simulink model "P3_SIM"  (R2024b)
settings: Solver=ode4  StartTime=0.0  StopTime=T_SIM  FixedStep=T_s  RelTol=1e-3
values from neighbouring files (symbols this model uses):
  D = diag([0.001, 0.001, 0.0175/6, 0.0175/6, 0.0175/6, 0.0175/6*T_s, 0.0175/6*T_s].^2)    [P3_script_FIXED.m]    (also in part3_results.mat = [1e-06 0 0 0 0 0 0 0 1e-06 0 0 0 ... (49 elements, 7x7)])
  d = 0.18428    [P3_script_FIXED.m]    (also in part3_results.mat)
  d_id = 0.18428    [P3_script_FIXED.m]    (also in part3_results.mat)
  H_enc = [0, 0, 0, 1, 0, 0, 0 ... (first row only)    [P3_script_FIXED.m]    (also in part3_results.mat = [0 0 0 0 0 0 1 0 0 1 0 0 ... (14 elements, 2x7)])
  H_gyro = [0, 0, 0, 0, 0, -r_id/d_id, r_id/d_id]    [P3_script_FIXED.m]    (also in part3_results.mat = [0 0 0 0 0 -0.179943564142 0.179943564142])
  H_motion_cap = [1, 0, 0, 0, 0, 0, 0 ... (first row only)    [P3_script_FIXED.m]    (also in part3_results.mat = [1 0 0 0 1 0 0 0 1 0 0 0 ... (21 elements, 3x7)])
  omega_max = 10    [P3_script_FIXED.m]    (also in part3_results.mat)
  P_INIT_EKF = diag([0.001, 0.001, 0.0175/6, 0.0175/6, 0.0175/6, 0.0175/6*T_s, 0.0175/6*T_s].^2)    [P3_script_FIXED.m]    (also in part3_results.mat = [1e-06 0 0 0 0 0 0 0 1e-06 0 0 0 ... (49 elements, 7x7)])
  p_loss = sim_output.p_loss.signals.values(1)    [P3_save_data.m]    (also in P3_script_FIXED.m = p_loss_values(i); part3_results.mat = 0)
  PHI_INIT = [0;0]    [P3_script_FIXED.m]    (also in part3_results.mat = [0 0])
  Q_INIT = q(:,1)    [P3_script_FIXED.m]    (also in part3_results.mat = [-0.5 -0.5 1.57079632679])
  Q_INIT_LOC = Q_INIT    [P3_script_FIXED.m]    (also in part3_results.mat = [-0.5 -0.5 1.57079632679])
  r = 0.03316    [P3_script_FIXED.m]    (also in part3_results.mat)
  R_3 = diag(([var_motion_capture, var_motion_capture, var_motion_capture,               ENCODER_QUANTIZATION/6, ENCODER_QUANTIZATION/6, var_IMU]).^2)    [P3_script_FIXED.m]    (also in part3_results.mat = [1e-06 0 0 0 0 0 0 1e-06 0 0 0 0 ... (36 elements, 6x6)])
  r_id = 0.03316    [P3_script_FIXED.m]    (also in part3_results.mat)
  T_s = (sim_output.tout(end)-sim_output.tout(1))/(length(sim_output.tout)-1)    [P3_save_data.m]    (also in P3_script_FIXED.m = 0.04; part3_results.mat = 0.04)
  Z_INIT_EKF = [Q_INIT; 0; 0; 0; 0]    [P3_script_FIXED.m]    (also in part3_results.mat = [-0.5 -0.5 1.57079632679 0 0 0 0])
undefined symbols (not defined in the file or in its folder): Ts, X, Y
libraries: robotlib x11, sharedtransform x1
settings Model: Creator=tomailoren  LastModifiedBy=tomailoren
settings OptimizationCC: DefaultParameterBehavior=Inlined  EnhancedBackFolding=on  PassReuseOutputArgsAs=Individual arguments  ZeroExternalMemoryAtStartup=off  ZeroInternalMemoryAtStartup=off  MaxStackSize=64  OptimizeBlockOrder=speed  DifferentSizesBufferReuse=on  OptimizationCustomize=off  EfficientTunableParamExpr=on
settings DebuggingCC: ParameterTunabilityLossMsg=error
settings HardwareCC: ProdBitPerPointer=32  ProdBitPerSizeT=32  ProdBitPerPtrDiffT=32  ProdLargestAtomicFloat=None  ProdIntDivRoundTo=Undefined  ProdEndianess=Unspecified  ProdWordSize=32  ProdHWDeviceType=Generic->Unspecified (assume 32-bit Generic)
settings SFSimCC: MATLABDynamicMemAlloc=off
settings RTWCC: Description=Embedded Coder  SystemTargetFile=ert.tlc  HardwareBoard=Robot Operating System (ROS)  TLCOptions="-aInlineSetEventsForThisBaseRateFcn=TLC_FALSE -aSuppressMultiTaskScheduler=TLC_FALSE  -aRateBasedStepFcn=0"  TemplateMakefile=ert_default_tmf  Toolchain=Catkin  TargetLang=C++
settings CodeAppCC: ForceParamTrailComments=on  IgnoreCustomStorageClasses=off  OperatorAnnotations=on  SimulinkDataObjDesc=on  SFDataObjDesc=on  InsertBlockDesc=on

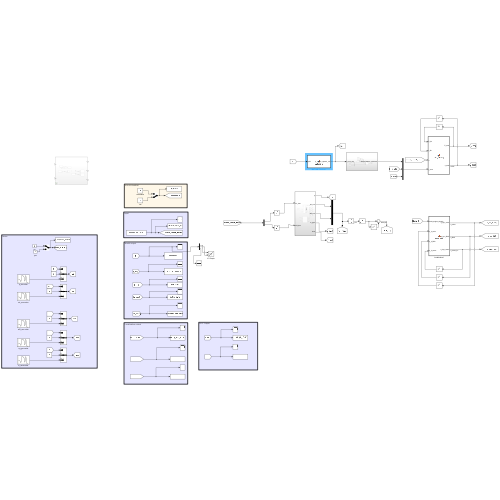
[thumbnail: Simulink's stored preview of the top-level diagram]
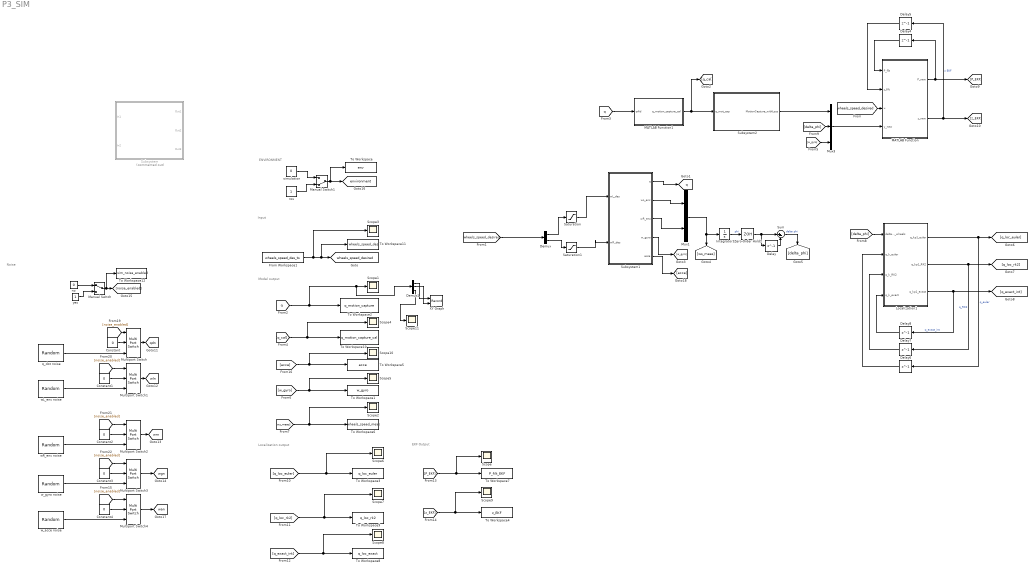
== system P3_SIM ==
  note: ENVIRONMENT
  note: Noise
  note: EKF Output
  note: Localization output
  note: Model output
  note: Input
  Constant{,1..4} (5 alike) : Constant  Value=0
  Delay : Delay  DelayLength=1  InitialCondition=[0;0]  SampleTime=T_s
  Delay4 : Delay  DelayLength=1  InitialCondition=P_INIT_EKF  SampleTime=T_s
  Delay5 : Delay  DelayLength=1  InitialCondition=Z_INIT_EKF  SampleTime=T_s
  Delay6 : Delay  DelayLength=1  InitialCondition=Q_INIT_LOC
  Delay7 : Delay  DelayLength=1  InitialCondition=Q_INIT_LOC
  Delay8 : Delay  DelayLength=1  InitialCondition=Q_INIT_LOC
  Demux : Demux  Outputs=2
  Demux1 : Demux  Outputs=3
  From Workspace1 : FromWorkspace  VariableName=wheels_speed_des_ts
  Integrator5 : Integrator  InitialCondition=PHI_INIT
  Localization1 : MATLAB Function  TreatAsAtomicUnit=on
  MATLAB Function : MATLAB Function  TreatAsAtomicUnit=on
  MATLAB Function1 : MATLAB Function  TreatAsAtomicUnit=on
  Manual Switch : ManualSwitch
  Manual Switch1 : ManualSwitch  CurrentSetting=0
  Multiport Switch{,1..4} (5 alike) : MultiPortSwitch  DataPortOrder=Zero-based contiguous  Inputs=2  zeroidx=on  SaturateOnIntegerOverflow=off  InputSameDT=off
  Mux1 : Mux  Inputs=2
  Mux3 : Mux  Inputs=3
  Saturation : Saturate  UpperLimit=omega_max  LowerLimit=-omega_max
  Saturation1 : Saturate  UpperLimit=omega_max  LowerLimit=-omega_max
  Scope{,1..11} (12 alike) : Scope
  Subsystem : Subsystem  Commented=on
  Subsystem1 : Subsystem
  Subsystem2 : Subsystem
  Sum : Sum  Inputs=|+-
  To Workspace : ToWorkspace  VariableName=env  SaveFormat=Structure  SampleTime=-1
      settings: Save2DSignal=2-D array (concatenate along first dimension)
  To Workspace1 : ToWorkspace  VariableName=w_gyro  SaveFormat=Structure With Time  SampleTime=-1
  To Workspace10 : ToWorkspace  VariableName=q_motion_capture_cal  SaveFormat=Structure With Time  SampleTime=-1
  To Workspace11 : ToWorkspace  VariableName=wheels_speed_des  SaveFormat=Structure With Time  SampleTime=-1
  To Workspace12 : ToWorkspace  VariableName=sim_noise_enabled  SaveFormat=Structure  SampleTime=-1
      settings: Save2DSignal=2-D array (concatenate along first dimension)
  To Workspace2 : ToWorkspace  VariableName=q_motion_capture  SaveFormat=Structure With Time  SampleTime=-1
  To Workspace3 : ToWorkspace  VariableName=q_loc_euler  SaveFormat=Structure With Time  SampleTime=-1
  To Workspace4 : ToWorkspace  VariableName=z_EKF  SaveFormat=Structure With Time  SampleTime=-1
  To Workspace5 : ToWorkspace  VariableName=acce  SaveFormat=Structure With Time  SampleTime=-1
  To Workspace6 : ToWorkspace  VariableName=wheels_speed_meas  SaveFormat=Structure With Time  SampleTime=-1
  To Workspace7 : ToWorkspace  VariableName=P_filt_EKF  SaveFormat=Structure With Time  SampleTime=-1
  To Workspace8 : ToWorkspace  VariableName=q_loc_exact  SaveFormat=Structure With Time  SampleTime=-1
  To Workspace9 : ToWorkspace  VariableName=q_loc_rk2  SaveFormat=Structure With Time  SampleTime=-1
  XY Graph : Record  FileSettingsInternal="{\"entries\":[{\"content\":{\"excelSettings\":{\"content\":{},\"type\":\"Streamout.ExcelSettings\"}},\"type\":\"Streamout.FileSettingStorage\",\"uuid\":\"\"}],\"packageUris\":[\"http:\\/\\/schema.mathworks.com\\/mf0\\/streamout_blocks\\/R2020a\"],\"version\":\"1.0\"}"  Layout=[1 1]  SignalsInternal="{\"entries\":[{\"content\":{\"signals\":[{\"content\":{\"blockPath\":[],\"dimensions\":[1,1],\"domain\":\"\",\"lineColor\":\"#a2142f\",\"plots\":[ 1 ],\"port\":1,\"sid\":[\"\"],\"signalID\":1,\"signalName\":\"Demux1:1\"},\"type\":\"RecordBlkView.Signal\",\"uuid\":\"\"},{\"content\":{\"blockPath\":[],\"dimensions\":[1,1],\"domain\":\"\",\"lineColor\":\"#139fff\",\"plots\":[ 1 ],\"port\":2,\"sid\":[\"\"],\"signalID\":2,\"signalName\":\"Demux1:2\"},\"type\":\"RecordBlkView.Signal\",\"uuid\":\"\"}]},\"type\":\"RecordBlkView.InputSignals\",\"uuid\":\"\"}],\"packageUris\":[\"http:\\/\\/schema.mathworks.com\\/mf0\\/streamout_blocks\\/R2020a\"],\"version\":\"1.0\"}"  VisualizationBindings="{\"xyplotplugin\":{\"info\":[{\"series\":[{\"bindingParametersList\":[{\"parameter\":\"X-Axis\",\"signalID\":1,\"signalName\":\"Demux1:1\"},{\"parameter\":\"Y-Axis\",\"signalID\":2,\"signalName\":\"Demux1:2\"}],\"seriesID\":0}],\"subplotID\":1}]}}"  CompatibilityTag=XY
  Zero-Order Hold1 : ZeroOrderHold  SampleTime=T_s
  no : Constant  Value=0
  q_dot noise : RandomNumber  SampleTime=T_s
  ros : Constant
  simulation : Constant  Value=0
  wL_enc noise : RandomNumber  Variance=0.25  Seed=1  SampleTime=T_s
  wR_enc noise : RandomNumber  Variance=0.25  Seed=2  SampleTime=T_s
  w_acce noise : RandomNumber  Variance=0.01  Seed=3  SampleTime=T_s
  w_gyro noise : RandomNumber  Variance=0.01  Seed=3  SampleTime=T_s
  yes : Constant
  tag scope: environment=global, q=global, qdn=global, wan=global, wgn=global, wheels_speed_desired=global, wln=global, wrn=global
  wires:
  Mux1/1 -> Integrator5/1, [ws_meas]
  Zero-Order Hold1/1 -> Delay/1, Sum/1
  Delay/1 -> Sum/2
  Integrator5/1 -> Zero-Order Hold1/1  "phi"
  Demux/1 -> Saturation/1
  Demux/2 -> Saturation1/1
  [wheels_speed_desired] -> Demux/1
  Delay5/1 -> MATLAB Function/2(z_filt)
  MATLAB Function/2(z_new) -> [z_EKF], Delay5/1  "z EKF"
  Delay4/1 -> MATLAB Function/1(P_filt)
  MATLAB Function/1(P_new) -> [P_EKF], Delay4/1
  Localization1/3(q_kp1_exact) -> [q_exact_int], Delay8/1  "q_exact_int"
  Localization1/1(q_kp1_euler) -> [q_loc_euler], Delay6/1  "q_euler"
  Delay6/1 -> Localization1/2(q_k_euler)
  Localization1/2(q_kp1_RK2) -> [q_loc_rk2], Delay7/1  "q_RK2"
  Delay8/1 -> Localization1/4(q_k_exact)
  Delay7/1 -> Localization1/3(q_k_RK2)
  Subsystem2/1(MotionCapture_withLoss) -> Mux3/1
  Mux3/1 -> MATLAB Function/4(y_new)
  MATLAB Function1/1(q_motion_capture_cal) -> [q_cal], Subsystem2/1(q_mot_cap)
  [wheels_speed_desired] -> MATLAB Function/3(u)
  From Workspace1/1 -> Scope3/1, To Workspace11/1, [wheels_speed_desired]
  [q] -> MATLAB Function1/1(q4id)
  [q_cal] -> To Workspace10/1, Scope4/1
  [w_gyro] -> Mux3/3
  [w_gyro] -> Scope5/1, To Workspace1/1
  [ws_meas] -> Scope2/1, To Workspace6/1
  Sum/1 -> [delta_phi]  "delta phi"
  [delta_phi] -> Localization1/1(delta_angles_wheels)
  [delta_phi] -> Mux3/2
  [q_loc_euler] -> Scope6/1, To Workspace3/1
  [q_loc_rk2] -> Scope7/1, To Workspace9/1
  [q_exact_int] -> Scope8/1, To Workspace8/1
  [P_EKF] -> Scope/1, To Workspace7/1
  [z_EKF] -> Scope9/1, To Workspace4/1
  Subsystem1/4(w_gyro) -> [w_gyro]
  Subsystem1/2(wL_enc) -> Mux1/1
  Subsystem1/3(wR_enc) -> Mux1/2
  yes/1 -> Manual Switch/2
  no/1 -> Manual Switch/1
  Manual Switch/1 -> To Workspace12/1, [noise_enabled]
  Multiport Switch/1 -> [qdn]
  [noise_enabled] -> Multiport Switch/1
  q_dot noise/1 -> Multiport Switch/3
  Constant/1 -> Multiport Switch/2
  [noise_enabled] -> Multiport Switch1/1
  Constant1/1 -> Multiport Switch1/2
  wL_enc noise/1 -> Multiport Switch1/3
  Multiport Switch1/1 -> [wln]
  [noise_enabled] -> Multiport Switch2/1
  Constant2/1 -> Multiport Switch2/2
  wR_enc noise/1 -> Multiport Switch2/3
  Multiport Switch2/1 -> [wrn]
  [noise_enabled] -> Multiport Switch3/1
  Constant3/1 -> Multiport Switch3/2
  Multiport Switch3/1 -> [wgn]
  w_gyro noise/1 -> Multiport Switch3/3
  Saturation/1 -> Subsystem1/1(wL_des)
  Saturation1/1 -> Subsystem1/2(wR_des)
  simulation/1 -> Manual Switch1/1
  ros/1 -> Manual Switch1/2
  Subsystem1/1(q) -> [q]
  Manual Switch1/1 -> To Workspace/1, [environment]
  Constant4/1 -> Multiport Switch4/2
  Multiport Switch4/1 -> [wan]
  w_acce noise/1 -> Multiport Switch4/3
  [noise_enabled] -> Multiport Switch4/1
  Subsystem1/5(acce) -> [acce]
  [acce] -> Scope10/1, To Workspace5/1
  [q] -> Demux1/1, Scope1/1, To Workspace2/1
  Demux1/3 -> Scope11/1
  Demux1/2 -> XY Graph/2
  Demux1/1 -> XY Graph/1

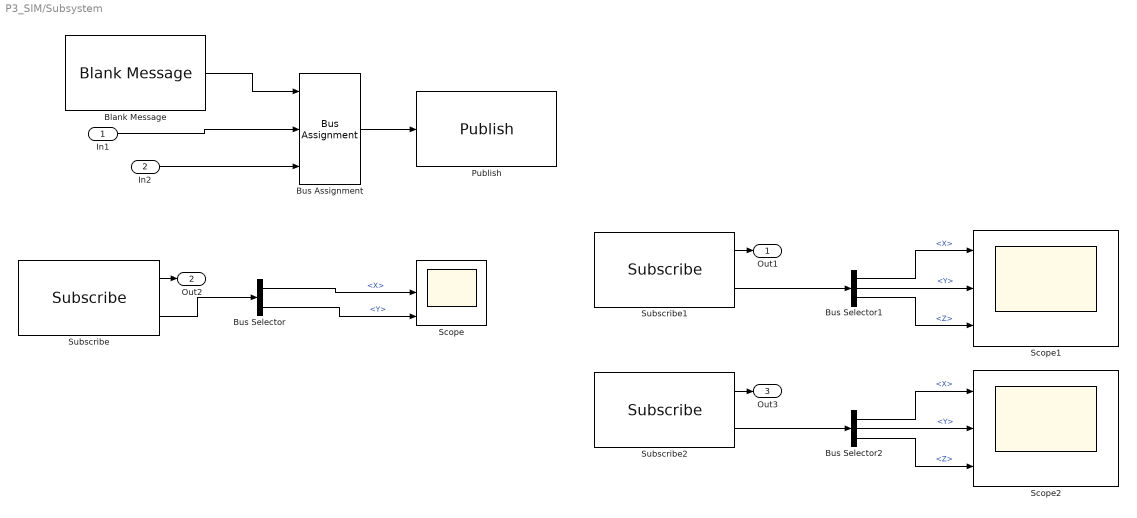
== system P3_SIM/Subsystem ==
  In1 : Inport
  In2 : Inport  Port=2
  Blank Message : robotlib/Blank Message  messageClass=Message  entityType=geometry_msgs/Vector3  messageType=geometry_msgs/Vector3  SampleTime=Ts  legacyBusStruct=off
  Bus Assignment : BusAssignment  AssignedSignals=X,Y
  Bus Selector : BusSelector  OutputSignals=X,Y
  Bus Selector1 : BusSelector  OutputSignals=X,Y,Z
  Bus Selector2 : BusSelector  OutputSignals=X,Y,Z
  Publish : robotlib/Publish  topicSource=Select from ROS network  topic=/turtlebot_01/cmd_wheels  messageType=geometry_msgs/Vector3  legacyBusStruct=off  messageQueueLength=1
  Scope : Scope  NumInputPorts=3
  Scope1 : Scope  NumInputPorts=3
  Scope2 : Scope  NumInputPorts=3
  Subscribe : robotlib/Subscribe  topicSource=Select from ROS network  topic=/turtlebot_01/wheelSpeeds  messageType=geometry_msgs/Vector3  SampleTime=Ts  legacyBusStruct=off  messageQueueLength=1
  Subscribe1 : robotlib/Subscribe  topicSource=Select from ROS network  topic=/turtlebot_01/gyroscope  messageType=geometry_msgs/Vector3  SampleTime=Ts  legacyBusStruct=off  messageQueueLength=1
  Subscribe2 : robotlib/Subscribe  topicSource=Select from ROS network  topic=/turtlebot_01/accelerometer  messageType=geometry_msgs/Vector3  SampleTime=Ts  legacyBusStruct=off  messageQueueLength=1
  Out1 : Outport
  Out2 : Outport  Port=2
  Out3 : Outport  Port=3
  wires:
  Bus Selector1/2 -> Scope1/2  "<Y>"
  Subscribe/2 -> Bus Selector/1
  Bus Selector2/1 -> Scope2/1  "<X>"
  Bus Selector1/3 -> Scope1/3  "<Z>"
  Bus Selector2/2 -> Scope2/2  "<Y>"
  Subscribe1/1 -> Out1/1
  Bus Assignment/1 -> Publish/1
  Bus Selector1/1 -> Scope1/1  "<X>"
  Bus Selector/1 -> Scope/2  "<X>"
  In2/1 -> Bus Assignment/3
  Subscribe1/2 -> Bus Selector1/1
  Subscribe2/2 -> Bus Selector2/1
  Blank Message/1 -> Bus Assignment/1
  Bus Selector/2 -> Scope/3  "<Y>"
  Bus Selector2/3 -> Scope2/3  "<Z>"
  In1/1 -> Bus Assignment/2
  Subscribe2/1 -> Out3/1
  Subscribe/1 -> Out2/1

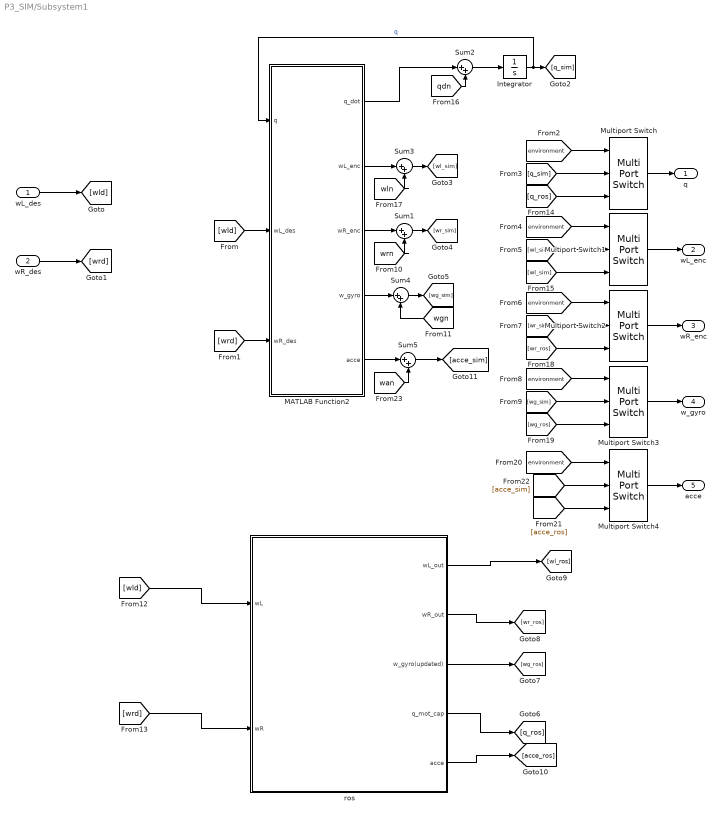
== system P3_SIM/Subsystem1 ==
  wL_des : Inport
  wR_des : Inport  Port=2
  Integrator : Integrator  InitialCondition=Q_INIT
  MATLAB Function2 : MATLAB Function  TreatAsAtomicUnit=on
  Multiport Switch{,1..4} (5 alike) : MultiPortSwitch  DataPortOrder=Zero-based contiguous  Inputs=2  zeroidx=on  SaturateOnIntegerOverflow=off  InputSameDT=off
  Sum{1..5} (5 alike) : Sum  Inputs=|++
  ros : Subsystem
  q : Outport
  wL_enc : Outport  Port=2
  wR_enc : Outport  Port=3
  w_gyro : Outport  Port=4
  acce : Outport  Port=5
  wires:
  Sum2/1 -> Integrator/1
  Integrator/1 -> [q_sim], MATLAB Function2/1(q)  "q"
  [qdn] -> Sum2/2
  MATLAB Function2/1(q_dot) -> Sum2/1
  wL_des/1 -> [wld]
  wR_des/1 -> [wrd]
  [wld] -> MATLAB Function2/2(wL_des)
  [wrd] -> MATLAB Function2/3(wR_des)
  [environment] -> Multiport Switch/1
  [q_sim] -> Multiport Switch/2
  Multiport Switch/1 -> q/1
  [environment] -> Multiport Switch1/1
  [wl_sim] -> Multiport Switch1/2
  Multiport Switch1/1 -> wL_enc/1
  [environment] -> Multiport Switch2/1
  [wr_sim] -> Multiport Switch2/2
  Multiport Switch2/1 -> wR_enc/1
  [environment] -> Multiport Switch3/1
  [wg_sim] -> Multiport Switch3/2
  Multiport Switch3/1 -> w_gyro/1
  [wln] -> Sum3/2
  Sum3/1 -> [wl_sim]
  MATLAB Function2/2(wL_enc) -> Sum3/1
  [wrn] -> Sum1/2
  MATLAB Function2/3(wR_enc) -> Sum1/1
  Sum1/1 -> [wr_sim]
  [wgn] -> Sum4/2
  MATLAB Function2/4(w_gyro) -> Sum4/1
  Sum4/1 -> [wg_sim]
  [q_ros] -> Multiport Switch/3
  [wl_sim] -> Multiport Switch1/3
  [wr_ros] -> Multiport Switch2/3
  [wg_ros] -> Multiport Switch3/3
  Multiport Switch4/1 -> acce/1
  [environment] -> Multiport Switch4/1
  [acce_sim] -> Multiport Switch4/2
  [acce_ros] -> Multiport Switch4/3
  MATLAB Function2/5(acce) -> Sum5/1
  Sum5/1 -> [acce_sim]
  [wan] -> Sum5/2
  ros/1(wL_out) -> [wl_ros]
  ros/2(wR_out) -> [wr_ros]
  ros/5(acce) -> [acce_ros]
  ros/4(q_mot_cap) -> [q_ros]
  ros/3(w_gyro(updated)) -> [wg_ros]
  [wld] -> ros/1(wL)
  [wrd] -> ros/2(wR)

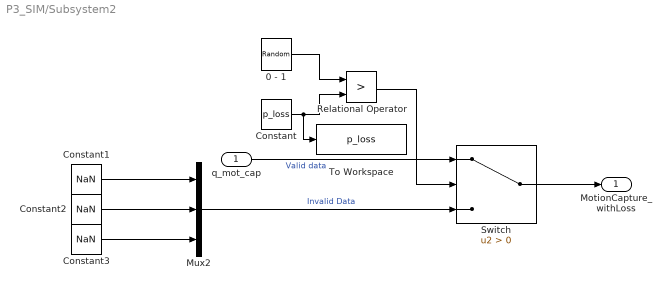
== system P3_SIM/Subsystem2 ==
  q_mot_cap : Inport
  0 - 1 : UniformRandomNumber  Minimum=0  SampleTime=T_s
  Constant : Constant  Value=p_loss
  Constant1 : Constant  Value=NaN
  Constant2 : Constant  Value=NaN
  Constant3 : Constant  Value=NaN
  Mux2 : Mux  Inputs=3
  Relational Operator : RelationalOperator  Operator=>  OutDataTypeStr=boolean  RndMeth=Simplest  InputSameDT=off
  Switch : Switch  Criteria=u2 > Threshold  SaturateOnIntegerOverflow=off  InputSameDT=off
  To Workspace : ToWorkspace  VariableName=p_loss  SaveFormat=Structure  SampleTime=-1
      settings: Save2DSignal=2-D array (concatenate along first dimension)
  MotionCapture_withLoss : Outport
  wires:
  0 - 1/1 -> Relational Operator/1
  Constant/1 -> To Workspace/1, Relational Operator/2
  Switch/1 -> MotionCapture_withLoss/1
  Relational Operator/1 -> Switch/2
  Constant2/1 -> Mux2/2
  Mux2/1 -> Switch/3  "Invalid Data"
  Constant1/1 -> Mux2/1
  q_mot_cap/1 -> Switch/1  "Valid data"
  Constant3/1 -> Mux2/3

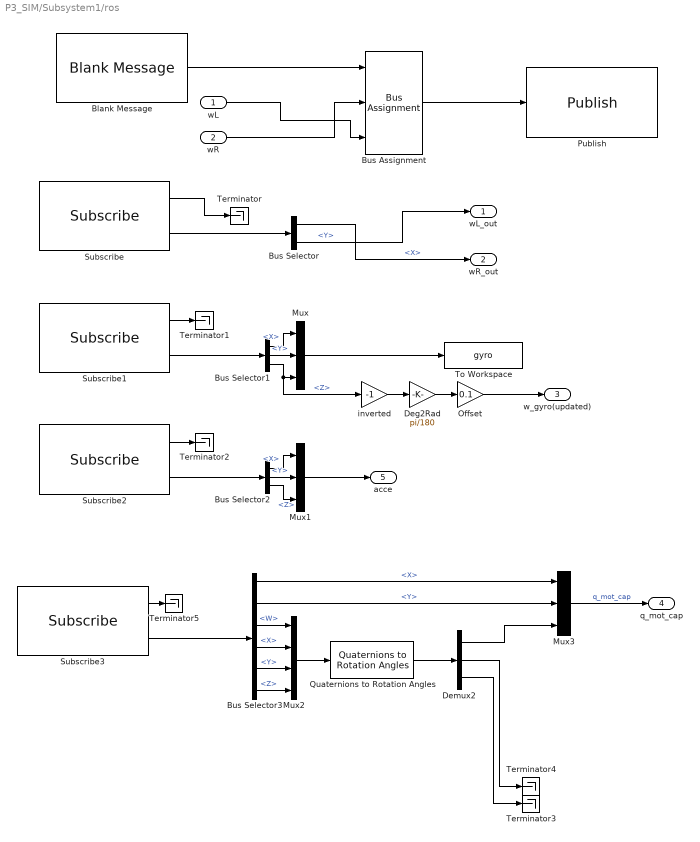
== system P3_SIM/Subsystem1/ros ==
  wL : Inport
  wR : Inport  Port=2
  Blank Message : robotlib/Blank Message  messageClass=Message  entityType=geometry_msgs/Vector3  messageType=geometry_msgs/Vector3  SampleTime=T_s  legacyBusStruct=off
  Bus Assignment : BusAssignment  AssignedSignals=X,Y
  Bus Selector : BusSelector  OutputSignals=X,Y
  Bus Selector1 : BusSelector  OutputSignals=X,Y,Z
  Bus Selector2 : BusSelector  OutputSignals=X,Y,Z
  Bus Selector3 : BusSelector  OutputSignals=Pose.Pose.Position.X,Pose.Pose.Position.Y,Pose.Pose.Orientation.W,Pose.Pose.Orientation.X,Pose.Pose.Orientation.Y,Pose.Pose.Orientation.Z
  Deg2Rad : Gain  Gain=pi/180
  Demux2 : Demux  Outputs=3
  Mux : Mux  Inputs=3
  Mux1 : Mux  Inputs=3
  Mux2 : Mux
  Mux3 : Mux  Inputs=3
  Offset : Gain  Gain=0.1
  Publish : robotlib/Publish  topicSource=Select from ROS network  topic=/turtlebot_01/cmd_wheels  messageType=geometry_msgs/Vector3  legacyBusStruct=off  messageQueueLength=1
  Quaternions to Rotation Angles : sharedtransform/Quaternions to Rotation Angles  rotationOrder=ZYX  aMode=aMode
  Subscribe : robotlib/Subscribe  topicSource=Select from ROS network  topic=/turtlebot_01/wheelSpeeds  messageType=geometry_msgs/Vector3  SampleTime=T_s  legacyBusStruct=off  messageQueueLength=1
  Subscribe1 : robotlib/Subscribe  topicSource=Select from ROS network  topic=/turtlebot_01/gyroscope  messageType=geometry_msgs/Vector3  SampleTime=T_s  legacyBusStruct=off  messageQueueLength=1
  Subscribe2 : robotlib/Subscribe  topicSource=Select from ROS network  topic=/turtlebot_01/accelerometer  messageType=geometry_msgs/Vector3  SampleTime=T_s  legacyBusStruct=off  messageQueueLength=1
  Subscribe3 : robotlib/Subscribe  topicSource=Select from ROS network  topic=/turtlebot_01/odom  messageType=nav_msgs/Odometry  SampleTime=T_s  legacyBusStruct=off  messageQueueLength=1
  Terminator{,1..5} (6 alike) : Terminator
  To Workspace : ToWorkspace  VariableName=gyro  SaveFormat=Structure With Time  SampleTime=-1
  inverted : Gain  Gain=-1
  wL_out : Outport
  wR_out : Outport  Port=2
  w_gyro(updated) : Outport  Port=3
  q_mot_cap : Outport  Port=4
  acce : Outport  Port=5
  wires:
  Subscribe2/2 -> Bus Selector2/1
  Bus Selector3/6 -> Mux2/4  "<Z>"
  Mux3/1 -> q_mot_cap/1  "q_mot_cap"
  wR/1 -> Bus Assignment/2
  Bus Selector/1 -> wR_out/1  "<X>"
  Bus Selector1/2 -> Mux/2  "<Y>"
  Bus Selector2/2 -> Mux1/2  "<Y>"
  Bus Selector2/1 -> Mux1/1  "<X>"
  Bus Assignment/1 -> Publish/1
  Subscribe2/1 -> Terminator2/1
  Demux2/2 -> Terminator4/1
  Mux2/1 -> Quaternions to Rotation Angles/1
  inverted/1 -> Deg2Rad/1
  Bus Selector3/4 -> Mux2/2  "<X>"
  Bus Selector3/1 -> Mux3/1  "<X>"
  Subscribe3/1 -> Terminator5/1
  Subscribe/2 -> Bus Selector/1
  Mux1/1 -> acce/1
  Deg2Rad/1 -> Offset/1
  Bus Selector3/5 -> Mux2/3  "<Y>"
  Quaternions to Rotation Angles/1 -> Demux2/1
  Bus Selector1/3 -> inverted/1, Mux/3  "<Z>"
  Demux2/3 -> Terminator3/1
  Demux2/1 -> Mux3/3
  Offset/1 -> w_gyro(updated)/1
  wL/1 -> Bus Assignment/3
  Bus Selector3/3 -> Mux2/1  "<W>"
  Bus Selector1/1 -> Mux/1  "<X>"
  Subscribe3/2 -> Bus Selector3/1
  Bus Selector2/3 -> Mux1/3  "<Z>"
  Mux/1 -> To Workspace/1
  Subscribe/1 -> Terminator/1
  Bus Selector/2 -> wL_out/1  "<Y>"
  Subscribe1/2 -> Bus Selector1/1
  Subscribe1/1 -> Terminator1/1
  Blank Message/1 -> Bus Assignment/1
  Bus Selector3/2 -> Mux3/2  "<Y>"

== matlab function P3_SIM/Localization1 ==
  data: delta_angles_wheels input; q_k_euler input; q_k_RK2 input; q_k_exact input; r_id parameter; d_id parameter; q_kp1_euler output; T_s parameter; q_kp1_RK2 output; q_kp1_exact output
function [q_kp1_euler, q_kp1_RK2, q_kp1_exact] = localization(delta_angles_wheels, q_k_euler, q_k_RK2, q_k_exact, r_id, d_id, T_s)

    r = r_id;
    d = d_id;

    % extraction data
    delta_phi_L = delta_angles_wheels(1);
    delta_phi_R = delta_angles_wheels(2);

    x_k_euler = q_k_euler(1); 
    y_k_euler = q_k_euler(2); 
    theta_k_euler = q_k_euler(3);
    
    x_k_RK2 = q_k_RK2(1); 
    y_k_RK2 = q_k_RK2(2); 
    theta_k_RK2 = q_k_RK2(3);

    x_k_exact = q_k_exact(1);
    y_k_exact = q_k_exact(2); 
    theta_k_exact = q_k_exact(3);


    % velocities estimate
    v_k = r / (2*T_s) * (delta_phi_R + delta_phi_L);
    w_k = r / (d*T_s) * (delta_phi_R - delta_phi_L);
    
    % Euler integration
    x_kp1_euler = x_k_euler + v_k * T_s * cos(theta_k_euler);
    y_kp1_euler = y_k_euler + v_k * T_s * sin(theta_k_euler);
    theta_kp1_euler = theta_k_euler + w_k * T_s;
    
    q_kp1_euler = [x_kp1_euler; y_kp1_euler; theta_kp1_euler];
    
    % RK2 Integration
    x_kp1_RK2 = x_k_RK2 + v_k * T_s * cos(theta_k_RK2 + (w_k * T_s)/2);
    y_kp1_RK2 = y_k_RK2 + v_k * T_s * sin(theta_k_RK2 + (w_k * T_s)/2);
    theta_kp1_RK2 = theta_k_RK2 + w_k * T_s;
    
    q_kp1_RK2 = [x_kp1_RK2; y_kp1_RK2; theta_kp1_RK2];
    
    % Exact Integration
    if abs(w_k) < 1e-4
        % use RK2 approximation to avoid division by zero when w_k is near 0
        x_kp1_exact = x_k_exact + v_k * T_s * cos(theta_k_exact + (w_k * T_s)/2);
        y_kp1_exact = y_k_exact + v_k * T_s * sin(theta_k_exact + (w_k * T_s)/2);
    else
        % Exact formulas
        x_kp1_exact = x_k_exact + (v_k / w_k) * (sin(theta_k_exact + w_k * T_s) - sin(theta_k_exact));
        y_kp1_exact = y_k_exact - (v_k / w_k) * (cos(theta_k_exact + w_k * T_s) - cos(theta_k_exact));
    end
    theta_kp1_exact = theta_k_exact + w_k * T_s;
    
    q_kp1_exact = [x_kp1_exact; y_kp1_exact; theta_kp1_exact];
    
end

== matlab function P3_SIM/MATLAB Function1 ==
  data: q4id input; q_motion_capture_cal output
function q_motion_capture_cal = calibration(q4id)

x_off_cal = -0.00434;
y_off_cal = -0.00361;
theta_off = 0.02331;


theta_cal = q4id(3) - theta_off;
x_cal = q4id(1) - (x_off_cal * cos(theta_cal) - y_off_cal * sin(theta_cal));
y_cal = q4id(2) - (x_off_cal * sin(theta_cal) + y_off_cal * cos(theta_cal));


q_motion_capture_cal = [x_cal; y_cal; theta_cal];

== matlab function P3_SIM/Subsystem1/MATLAB Function2 ==
  data: q input; q_dot output; wL_des input; wR_des input; wL_enc output; wR_enc output; w_gyro output; r parameter; d parameter; T_s parameter; acce output
function [q_dot, wL_enc, wR_enc, w_gyro, acce] = robot_simulator(q, wL_des, wR_des, r, d, T_s)
    
    wL_enc = wL_des;
    wR_enc = wR_des;
      
    v = (r/2) * (wR_des + wL_des);
    omega = (r/d) * (wR_des - wL_des);
    
    w_gyro = -omega;
    
    q_dot= zeros(3,1);
    
    q_dot(1) = v*cos(q(3));
    q_dot(2) = v*sin(q(3));
    q_dot(3) = omega;

    acce = [0;0;0];
    
end

== matlab function P3_SIM/MATLAB Function ==
  data: P_filt input; P_new output; z_filt input; z_new output; u input; y_new input; D parameter; T_s parameter; r_id parameter; d_id parameter; H_enc parameter; H_gyro parameter; H_motion_cap parameter; R_3 parameter
function [P_new, z_new] = EKF_filtering(P_filt, z_filt, u, y_new, D, T_s, r_id, d_id, H_enc, H_gyro, H_motion_cap, R_3)

    % Def state z_filt: [xk , yk , thetak , delta_phi_L_km1 , delta_phi_R_km1 , wLk , wRk ]

    r = r_id;
    d = d_id;
        
    % Extraction variables
    x_k = z_filt(1);
    y_k = z_filt(2);
    theta_k = z_filt(3);
    delta_phi_L_km1 = z_filt(4);
    delta_phi_R_km1 = z_filt(5); 
    wL_k = z_filt(6);               % estimate wheels velocities
    wR_k = z_filt(7);
    
    uL_k = u(1);                    % actual wheels velocities (from command input v,w)
    uR_k = u(2);

    % ----------------------

    % PREDICT STEP
    v_k = (r/2) * (wL_k + wR_k);
    omega_k = (r/d) * (wR_k - wL_k);
    theta_mean = theta_k + (omega_k * T_s) / 2;
        
    % State Prediction (approximation with RK2)
    x_kp1 = x_k + v_k * T_s * cos(theta_mean);
    y_kp1 = y_k + v_k * T_s * sin(theta_mean);
    theta_kp1 = theta_k + omega_k * T_s;
    
    delta_phi_L_k = wL_k * T_s;
    delta_phi_R_k = wR_k * T_s;
    
    wL_kp1 = uL_k; 
    wR_kp1 = uR_k;
    
    z_hat = [x_kp1; y_kp1; theta_kp1; delta_phi_L_k; delta_phi_R_k; wL_kp1; wR_kp1];
    
    % F derivation
    F = zeros(7,7);
    
    F(1,1) = 1;
    F(1, 3) = -T_s * v_k * sin(theta_mean);
    F(1, 6) = (T_s * r / 2) * cos(theta_mean) - v_k * T_s * sin(theta_mean) * (-T_s * r / (2 * d));
    F(1, 7) = (T_s * r / 2) * cos(theta_mean) - v_k * T_s * sin(theta_mean) * (T_s * r / (2 * d));
    
    F(2,2) = 1;
    F(2, 3) = v_k * T_s * cos(theta_mean);
    F(2, 6) = (T_s * r / 2) * sin(theta_mean) + v_k * T_s * cos(theta_mean) * (-T_s * r / (2 * d));
    F(2, 7) = (T_s * r / 2) * sin(theta_mean) + v_k * T_s * cos(theta_mean) * (T_s * r / (2 * d));

    F(3,3) = 1;
    F(3, 6) = -T_s * r / d;
    F(3, 7) = T_s * r / d;

    F(4, 6) = T_s;
    F(5, 7) = T_s;
    
    % Covariance Prediction
    P_hat = F * P_filt * F' + D;
    
    % ----------------------

    % UPDATE STEP
    % H and R will depend on the measurement data y_new and Test_case

    % enc_values (delta_phi)
    % IMU_values (w_gyro)
    % Motion_capture (state q)

    % y_new = [x; y; theta; delta_phi_L; delta_phi_R; omega_gyro]

    %% OBSERVATION MATRIX H ALWAYS FULL (6X7) AND ALSO Y_NEW (6X1) 
    H_full = [H_motion_cap; H_enc; H_gyro];
    y_meas = y_new; 
    
    % Usiamo la R_3 (6x6) come base
    R_current = R_3;
    INFINITY_VAR = 1e9; % Incertezza "infinita" per spegnere il Kalman Gain
    
    % TEST 3: Tutti attivi, perdita pacchetto Mocap dinamica
    if any(isnan(y_new(1:3)))
        y_meas(1:3) = 0; % Mocap perso -> forziamo a zero
        R_current(1,1) = INFINITY_VAR; R_current(2,2) = INFINITY_VAR; R_current(3,3) = INFINITY_VAR;
    end

    
    % Innovation e_pred
    y_hat = H_full * z_hat;
    e_kp1 = y_meas - y_hat;
    
    % Kalman Gain K_pred
    K = P_hat * H_full' / (H_full * P_hat * H_full' + R_current);   
    
    % State and Covariance Update
    z_new = z_hat + K * e_kp1;
    P_new = P_hat - K * H_full * P_hat;


end
